simulink model "Example_SS_Exciter_Rogers"  (R2023a)
settings: Solver=ode45  StartTime=0.0  StopTime=20  RelTol=1e-3
undefined symbols (not defined in the file): K, Kf, Ta, Tb, Tc, Tf, Tr
settings Model: Creator=fglon  LastModifiedBy=fglon
settings ModelReferenceCC: EnableRefExpFcnMdlSchedulingChecks=on

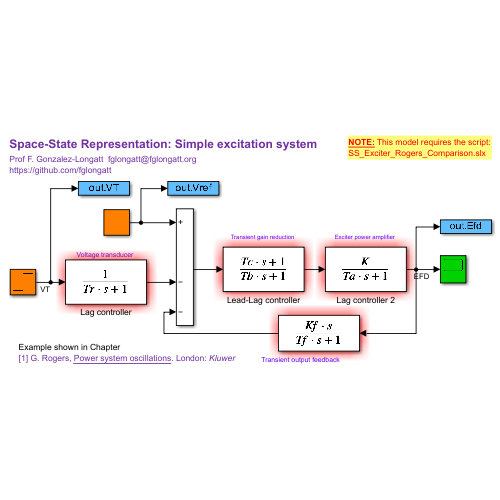
[thumbnail: Simulink's stored preview of the top-level diagram]
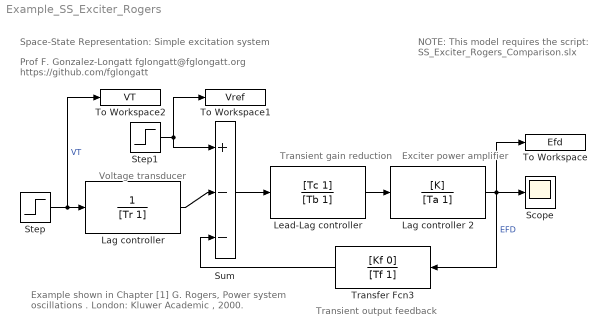
== system Example_SS_Exciter_Rogers ==
  note: NOTE: This model requires the script:
      | SS_Exciter_Rogers_Comparison.slx
  note: Voltage transducer
  note: Transient output feedback
  note: Exciter power amplifier
  note: Transient gain reduction
  note: Prof F. Gonzalez-Longatt fglongatt@fglongatt.org
      | https://github.com/fglongatt
  note: Space-State Representation: Simple excitation system
  note: Example shown in Chapter
      | [1] G. Rogers, Power system oscillations . London: Kluwer Academic , 2000.
  "Lag controller " : TransferFcn  Denominator=[Tr 1]
  Lag controller 2 : TransferFcn  Numerator=[K]  Denominator=[Ta 1]
  "Lead-Lag controller " : TransferFcn  Numerator=[Tc 1]  Denominator=[Tb 1]
  Scope : Scope
  Step : Step  Time=0  SampleTime=0
  Step1 : Step  Time=100  SampleTime=0
  Sum : Sum  Inputs=+|--
  To Workspace : ToWorkspace  VariableName=Efd  SaveFormat=Timeseries  SampleTime=-1
  To Workspace1 : ToWorkspace  VariableName=Vref  SaveFormat=Timeseries  SampleTime=-1
  To Workspace2 : ToWorkspace  VariableName=VT  SaveFormat=Timeseries  SampleTime=-1
  Transfer Fcn3 : TransferFcn  Numerator=[Kf 0]  Denominator=[Tf 1]
  wires:
  Lag controller 2/1 -> To Workspace/1, Transfer Fcn3/1, Scope/1  "EFD"
  "Lead-Lag controller "/1 -> Lag controller 2/1
  Sum/1 -> "Lead-Lag controller "/1
  Step/1 -> To Workspace2/1, "Lag controller "/1  "VT"
  Transfer Fcn3/1 -> Sum/3
  "Lag controller "/1 -> Sum/2
  Step1/1 -> To Workspace1/1, Sum/1
